simulink model "Sim38"  (R2019a)
settings: Solver=FixedStepAuto  StartTime=0.0  StopTime=10.0  FixedStep=0.0001  RelTol=1e-3
settings Model: Creator=fbleo  LastModifiedBy=fbleo

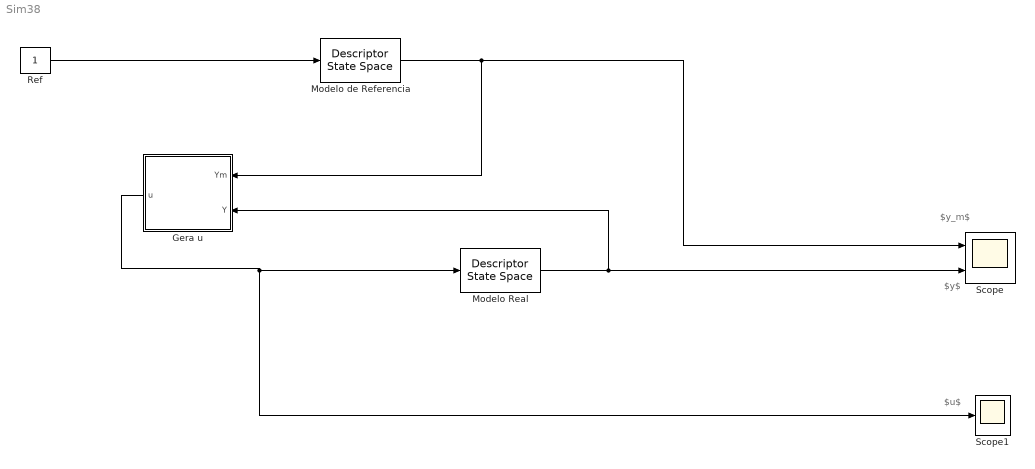
== system Sim38 ==
  note: $u$
  note: $y$
  note: $y_m$
  Gera u : Subsystem
  Modelo Real : DescriptorStateSpace  A=-1  B=2  D=0  InitialCondition=0.5
  Modelo de Referencia : DescriptorStateSpace  A=-3  B=3  D=0  InitialCondition=0
  Ref : Constant
  Scope : Scope  NumInputPorts=2
  Scope1 : Scope
  wires:
  Ref/1 -> Modelo de Referencia/1
  Modelo Real/1 -> Scope/2, Gera u/2(Y)
  Gera u/1(u) -> Modelo Real/1, Scope1/1
  Modelo de Referencia/1 -> Scope/1, Gera u/1(Ym)

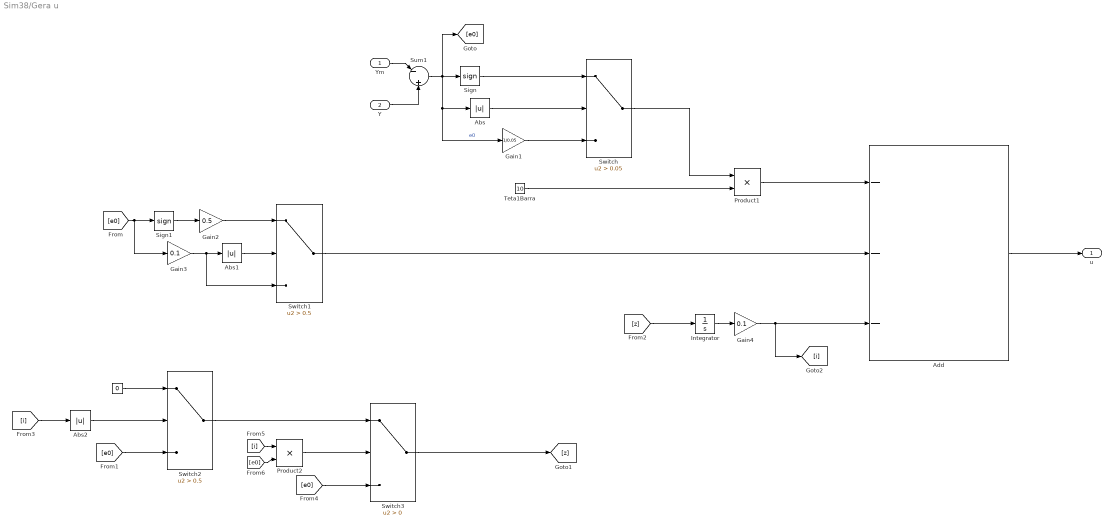
== system Sim38/Gera u ==
  Ym : Inport
  Y : Inport  Port=2
  " " : Constant  Value=0
  Abs : Abs
  Abs1 : Abs
  Abs2 : Abs
  Add : Sum  Inputs=---
  Gain1 : Gain  Gain=1/0.05
  Gain2 : Gain  Gain=0.5
  Gain3 : Gain  Gain=0.1
  Gain4 : Gain  Gain=0.1
  Integrator : Integrator
  Product1 : Product
  Product2 : Product
  Sign : Signum
  Sign1 : Signum
  Sum1 : Sum  Inputs=|-||+
  Switch : Switch  Criteria=u2 > Threshold  Threshold=0.05
  Switch1 : Switch  Criteria=u2 > Threshold  Threshold=0.5
  Switch2 : Switch  Criteria=u2 > Threshold  Threshold=0.5
  Switch3 : Switch  Criteria=u2 > Threshold
  Teta1Barra : Constant  Value=10
  u : Outport
  wires:
  Ym/1 -> Sum1/1
  Y/1 -> Sum1/2
  Teta1Barra/1 -> Product1/2
  Switch/1 -> Product1/1
  Sign/1 -> Switch/1
  Sum1/1 -> [e0], Gain1/1, Abs/1, Sign/1  "e0"
  Abs/1 -> Switch/2
  Gain1/1 -> Switch/3
  Product1/1 -> Add/1
  [e0] -> Gain3/1, Sign1/1
  Sign1/1 -> Gain2/1
  Gain2/1 -> Switch1/1
  Gain3/1 -> Switch1/3, Abs1/1
  Abs1/1 -> Switch1/2
  Switch1/1 -> Add/2
  [e0] -> Switch2/3
  " "/1 -> Switch2/1
  Switch2/1 -> Switch3/1
  [z] -> Integrator/1
  Integrator/1 -> Gain4/1
  Gain4/1 -> [i], Add/3
  [i] -> Abs2/1
  Abs2/1 -> Switch2/2
  Switch3/1 -> [z]
  [e0] -> Switch3/3
  [i] -> Product2/1
  [e0] -> Product2/2
  Product2/1 -> Switch3/2
  Add/1 -> u/1
